simulink model "RCAM_SimulinkModel"  (R2022b)
settings: Solver=VariableStepAuto  StartTime=0.0  StopTime=TF  RelTol=1e-3
values from neighbouring files (symbols this model uses):
  U0 = [0 ... (first row only)    [RCAM_model_initialConditions.m]    (also in designPIL.m)
  X0 = [100 ... (first row only)    [RCAM_model_initialConditions.m]    (also in designPIL.m = [85)
undefined symbols (not defined in the file or in its folder): RCAM_model
settings Model: Creator=bendr  LastModifiedBy=bendr

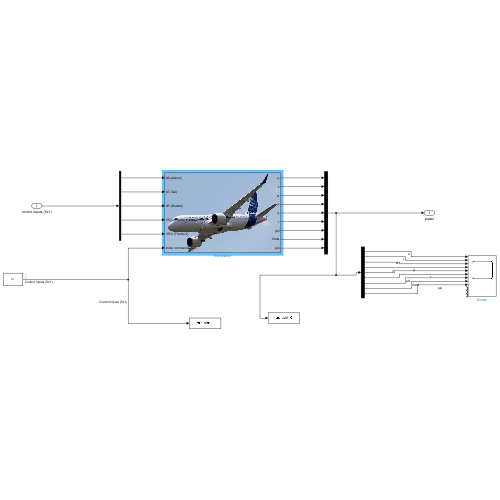
[thumbnail: Simulink's stored preview of the top-level diagram]
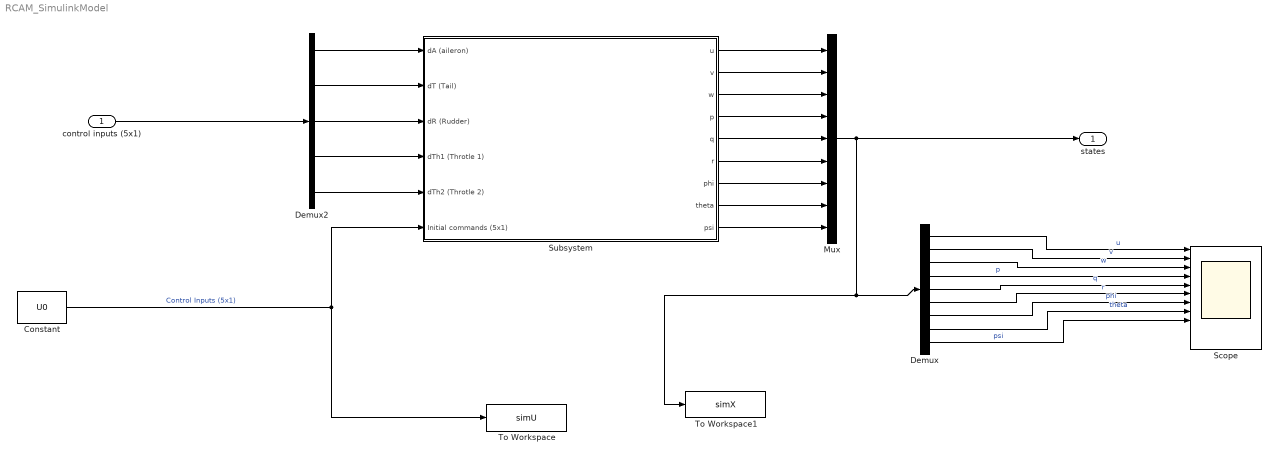
== system RCAM_SimulinkModel ==
  control inputs (5x1) : Inport
  Constant : Constant  Value=U0
  Demux : Demux  Outputs=9
  Demux2 : Demux  Outputs=5
  Mux : Mux  Inputs=9
  Scope : Scope  NumInputPorts=12
  Subsystem : Subsystem
      mask Display: image('C:\Users\bendr\OneDrive - ISAE-SUPAERO\AFCS\Aircraft_model\airbus.webp'); % Use "Edit Image" on toolstrip to change.
  To Workspace : ToWorkspace  VariableName=simU  SaveFormat=Timeseries  SampleTime=-1
  To Workspace1 : ToWorkspace  VariableName=simX  SaveFormat=Timeseries  SampleTime=-1
  states : Outport
  wires:
  Constant/1 -> To Workspace/1, Subsystem/6(Initial commands (5x1))  "Control Inputs (5x1)"
  Demux/2 -> Scope/2  "v"
  Demux/1 -> Scope/1  "u"
  Demux/3 -> Scope/3  "w"
  Demux/4 -> Scope/4  "p"
  Demux/5 -> Scope/5  "q"
  Demux/6 -> Scope/6  "r"
  Demux/7 -> Scope/7  "phi"
  Demux/8 -> Scope/8  "theta"
  Demux/9 -> Scope/9  "psi"
  Demux2/3 -> Subsystem/3(dR (Rudder))
  Demux2/4 -> Subsystem/4(dTh1 (Throtle 1))
  Demux2/5 -> Subsystem/5(dTh2 (Throtle 2))
  Demux2/2 -> Subsystem/2(dT (Tail))
  Demux2/1 -> Subsystem/1(dA (aileron))
  Subsystem/1(u) -> Mux/1
  Subsystem/2(v) -> Mux/2
  Subsystem/3(w) -> Mux/3
  Subsystem/4(p) -> Mux/4
  Subsystem/5(q) -> Mux/5
  Subsystem/6(r) -> Mux/6
  Subsystem/7(phi) -> Mux/7
  Subsystem/8(theta) -> Mux/8
  Mux/1 -> To Workspace1/1, Demux/1, states/1
  Subsystem/9(psi) -> Mux/9
  control inputs (5x1)/1 -> Demux2/1

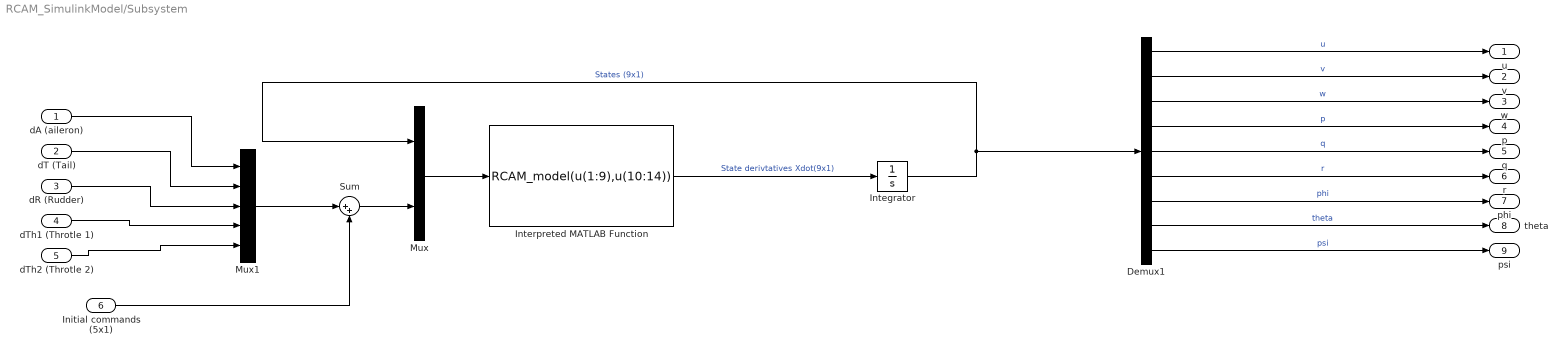
== system RCAM_SimulinkModel/Subsystem ==
  dA (aileron) : Inport
  dT (Tail) : Inport  Port=2
  dR (Rudder) : Inport  Port=3
  dTh1 (Throtle 1) : Inport  Port=4
  dTh2 (Throtle 2) : Inport  Port=5
  Initial commands (5x1) : Inport  Port=6
  Demux1 : Demux  Outputs=9
  Integrator : Integrator  InitialCondition=X0
  Interpreted MATLAB Function : MATLABFcn  MATLABFcn=RCAM_model(u(1:9),u(10:14))
  Mux : Mux  Inputs=2
  Mux1 : Mux  Inputs=5
  Sum : Sum  Inputs=|++
  u : Outport
  v : Outport  Port=2
  w : Outport  Port=3
  p : Outport  Port=4
  q : Outport  Port=5
  r : Outport  Port=6
  phi : Outport  Port=7
  theta : Outport  Port=8
  psi : Outport  Port=9
  wires:
  Interpreted MATLAB Function/1 -> Integrator/1  "State derivtatives Xdot(9x1)"
  Mux/1 -> Interpreted MATLAB Function/1
  Integrator/1 -> Mux/1, Demux1/1  "States (9x1)"
  Demux1/8 -> theta/1  "theta"
  Demux1/6 -> r/1  "r"
  Demux1/9 -> psi/1  "psi"
  Demux1/2 -> v/1  "v"
  Demux1/7 -> phi/1  "phi"
  Demux1/1 -> u/1  "u"
  Demux1/5 -> q/1  "q"
  Demux1/4 -> p/1  "p"
  Demux1/3 -> w/1  "w"
  Sum/1 -> Mux/2
  Initial commands (5x1)/1 -> Sum/2
  dR (Rudder)/1 -> Mux1/3
  dTh2 (Throtle 2)/1 -> Mux1/5
  dT (Tail)/1 -> Mux1/2
  dTh1 (Throtle 1)/1 -> Mux1/4
  dA (aileron)/1 -> Mux1/1
  Mux1/1 -> Sum/1
